simulink model "mathematical_modeling3"  (R2017b)
settings: Solver=VariableStepAuto  StartTime=0.0  StopTime=10  RelTol=1e-3
values from neighbouring files (symbols this model uses):
  k1 = 5    [mathematical_modeling2_parameters.m]    (also in mathematical_modeling3_parameters.m)
  k2 = 5    [mathematical_modeling2_parameters.m]    (also in mathematical_modeling3_parameters.m)
  k3 = 5    [mathematical_modeling2_parameters.m]    (also in mathematical_modeling3_parameters.m)
  m1 = 1    [mathematical_modeling2_parameters.m]    (also in mathematical_modeling3_parameters.m)
  m2 = 3    [mathematical_modeling2_parameters.m]    (also in mathematical_modeling3_parameters.m)
settings Model: Creator=Damla  LastModifiedBy=dagac

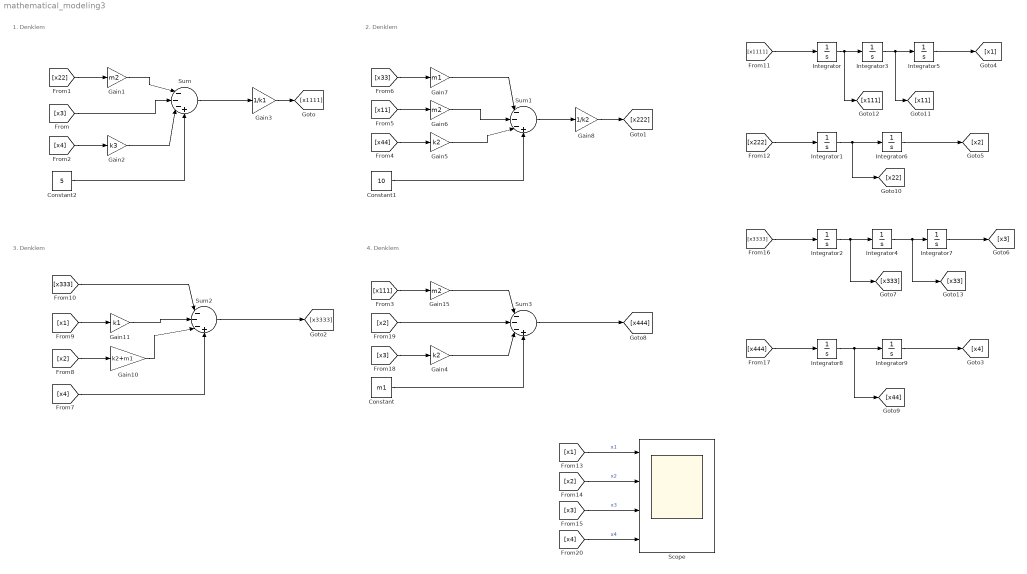
== system mathematical_modeling3 ==
  note: 1. Denklem
  note: 2. Denklem
  note: 3. Denklem
  note: 4. Denklem
  Constant : Constant  Value=m1
  Constant1 : Constant  Value=10
  Constant2 : Constant  Value=5
  Gain1 : Gain  Gain=m2
  Gain10 : Gain  Gain=k2+m1
  Gain11 : Gain  Gain=k1
  Gain15 : Gain  Gain=m2
  Gain2 : Gain  Gain=k3
  Gain3 : Gain  Gain=1/k1
  Gain4 : Gain  Gain=k2
  Gain5 : Gain  Gain=k2
  Gain6 : Gain  Gain=m2
  Gain7 : Gain  Gain=m1
  Gain8 : Gain  Gain=1/k2
  Integrator{,1..9} (10 alike) : Integrator
  Scope : Scope  NumInputPorts=4
  Sum{,1..3} (4 alike) : Sum  Inputs=|---+
  wires:
  Gain1/1 -> Sum/1
  [x4] -> Sum2/4
  [x2] -> Gain10/1
  Gain11/1 -> Sum2/2
  Gain10/1 -> Sum2/3
  [x3] -> Sum/2
  [x333] -> Sum2/1
  [x2] -> Scope/2  "x2"
  Integrator1/1 -> [x22], Integrator6/1
  [x1] -> Scope/1  "x1"
  [x33] -> Gain7/1
  Gain7/1 -> Sum1/1
  Gain5/1 -> Sum1/3
  [x222] -> Integrator1/1
  [x44] -> Gain5/1
  Gain6/1 -> Sum1/2
  [x3333] -> Integrator2/1
  [x3] -> Scope/3  "x3"
  [x1] -> Gain11/1
  Gain2/1 -> Sum/3
  Integrator2/1 -> [x333], Integrator4/1
  Gain3/1 -> [x1111]
  Gain8/1 -> [x222]
  [x1111] -> Integrator/1
  [x4] -> Gain2/1
  Integrator/1 -> [x111], Integrator3/1
  [x11] -> Gain6/1
  Sum1/1 -> Gain8/1
  [x22] -> Gain1/1
  Sum/1 -> Gain3/1
  Integrator3/1 -> [x11], Integrator5/1
  Sum2/1 -> [x3333]
  Integrator4/1 -> [x33], Integrator7/1
  Constant2/1 -> Sum/4
  Constant1/1 -> Sum1/4
  Sum3/1 -> [x444]
  Gain4/1 -> Sum3/3
  [x111] -> Gain15/1
  [x3] -> Gain4/1
  [x2] -> Sum3/2
  Gain15/1 -> Sum3/1
  Integrator5/1 -> [x1]
  Integrator6/1 -> [x2]
  Integrator7/1 -> [x3]
  Integrator8/1 -> [x44], Integrator9/1
  [x444] -> Integrator8/1
  Integrator9/1 -> [x4]
  Constant/1 -> Sum3/4
  [x4] -> Scope/4  "x4"
